simulink model "sedemo_rateestimator_withidlecomp"  (Simulink 7.5)
settings: Solver=VariableStepDiscrete  StartTime=0.0  StopTime=1200  MaxStep=inf  RelTol=1e-3
libraries: simeventssink1 x6, simeventstranslate1 x3, simeventsrouting1 x2, simeventstiming1 x2, simeventsgenerators1 x2, simeventsgates1 x1, simeventsqueue1 x1, simeventsinfo x1, simulink x1
settings Model: Creator=The MathWorks Inc.
settings DataIOCC: SaveOutput=off  SaveTime=off
settings OptimizationCC: InitFltsAndDblsToZero=on  EfficientMapNaN2IntZero=off
settings DebuggingCC: AlgebraicLoopMsg=error  SolverPrmCheckMsg=none  StrictBusMsg=Warning
settings SimEventsCC: propDiagAttribOutput=1  propDiagFcnCallOutput=1  propDiagStatOutput=0

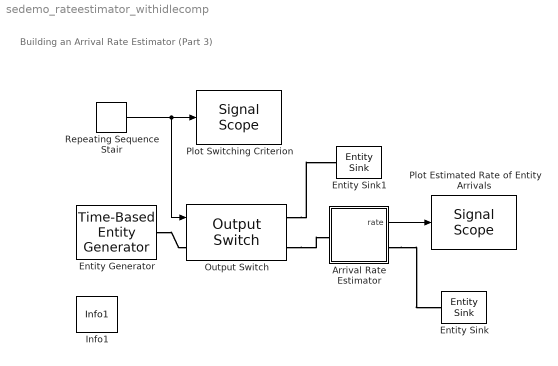
== system sedemo_rateestimator_withidlecomp ==
  note: Building an Arrival Rate Estimator (Part 3)
  Arrival Rate Estimator : Subsystem  mask(Rate Estimator){p=0.1, t_def=30}
      mask prompts: p "Smoothing factor p (0<p<1):"; t_def "Default sampling interval:"
      mask help:
      | Estimate number of arriving entities per second, where p is a smoothing factor that determines how much weight is given to the old estimate. If p is near 0, the estimate is more sensitive. If p is near 1, the estimate is smoother.
      |
      | The default sampling interval indicates the period of rate estimation computations during idle intervals when no entities arrive.
  Entity Generator : simeventsgenerators1/Entity Generators/Time-Based Entity Generator  Priority=1  DialogController=des_ddg_create  DialogControllerArgs=DataTag13  SystemSampleTime=-1  GenerateEntitiesUpon=Intergeneration time from dialog  Distribution=Constant  Minimum=0  Maximum=1  Mean=1  InitialSeed=12345  Period=4  PriorityEntityGeneration=300  GenerateEntityAtSimulationStart=off  ResponseWhenBlocked=Pause generation  ResponseWhenUnblocked=Immediate restart  EntityType=Standard  StatNumberDeparted=Off  StatPendingEntity=Off  StatAverageIntergenerationTime=Off
      settings: AttributesFormatString=Period = %<Period>
  Entity Sink : simeventssink1/Entity Sink  Priority=1  SystemSampleTime=-1  AvailableForArrivals=on  StatNumberArrived=Off
  Entity Sink1 : simeventssink1/Entity Sink  Priority=1  SystemSampleTime=-1  AvailableForArrivals=on  StatNumberArrived=Off
  Info1 : simeventsinfo/Info1  SystemSampleTime=-1  file_name=sedemo_rateestimator_m
  Output Switch : simeventsrouting1/Output Switch  Priority=1  SystemSampleTime=-1  NumberOutputPorts=2  SwitchingCriterion=From signal port p  InitialSeed=34567  AttributeName=Attribute1  InitialConditionsOpt=on  InitialConditions=1  EntityBufferOpt=off  SpecifyEventPriority=off  PriorityOutputSwitchSelectPort=4100  TimeoutPortOpt=off  StatNumberDeparted=Off  StatNumberTimedOut=Off  StatPendingEntity=Off  StatLastDeparturePort=Off  EvaluatedNumPorts=2
  Plot Estimated Rate of Entity Arrivals : simeventssink1/Signal Scope  Priority=1  SystemSampleTime=-1  PlotType=Continuous  InputType=Signal  NumInputs=1  AttributeNameY=Count  XInputOptionSignal=Event time  XInputOptionEntity=Event time  AttributeNameX=Count  EnableEntityOutport=on  XMin=-3  XMax=1203  XLimitExceededOption=Stretch axis limits  YLimitExceededOption=Stretch axis limits  AxisGrid=on  AxisLegend=off  LineDisables=""  LineColors="0  0  1"  LineStyles=-  LineMarkers=.  OpenScopeAtSimStart=on  Title=Arrival Rate Estimated Upon Arrivals and During Idle Intervals  YLabel=""  XLabel=Time  FigurePosition=[517 203 438 210]  AxisZoom=off  DataStoreOption=Limited  DataPointsLimit=10000  StatNumberArrived=Off  ShowCountPlotted=off  ShowToolbar=on
      settings: YMin=-0.005  YMax=.3
  Plot Switching Criterion : simeventssink1/Signal Scope  Priority=1  SystemSampleTime=-1  PlotType=Stair  InputType=Signal  NumInputs=1  AttributeNameY=Count  XInputOptionSignal=Event time  XInputOptionEntity=Event time  AttributeNameX=Count  EnableEntityOutport=on  XMin=-3  XMax=1203  XLimitExceededOption=Stretch axis limits  YLimitExceededOption=Keep axis limits unchanged  AxisGrid=off  AxisLegend=off  LineDisables=""  LineColors="1  0  0"  LineStyles=-  LineMarkers=.  OpenScopeAtSimStart=off  Title=Switching Criterion (p=2 is through rate estimator)  YLabel=""  XLabel=Time  FigurePosition=[517 488 438 210]  AxisZoom=off  DataStoreOption=Limited  DataPointsLimit=10000  StatNumberArrived=Off  ShowCountPlotted=off  ShowToolbar=on
      settings: YMin=0.9  YMax=2.1
  Repeating Sequence Stair : simulink/Sources/Repeating Sequence Stair  SystemSampleTime=-1  OutValues=[2 1 2 1]  tsamp=200  OutMin=[]  OutMax=[]  OutDataTypeStr=float('double')  OutputDataTypeScalingMode=Specify via dialog  OutDataType=float('double')  ConRadixGroup=Best Precision: Vector-wise  OutScaling=2^-12
  wires:
  Arrival Rate Estimator/1(rate) -> Plot Estimated Rate of Entity Arrivals/1
  Repeating Sequence Stair/1 -> Output Switch/1, Plot Switching Criterion/1
  connections:
  Entity Generator/RConn1 -- Output Switch/LConn1
  Output Switch/RConn1 -- Entity Sink1/LConn1
  Output Switch/RConn2 -- Arrival Rate Estimator/LConn1
  Arrival Rate Estimator/RConn1 -- Entity Sink/LConn1

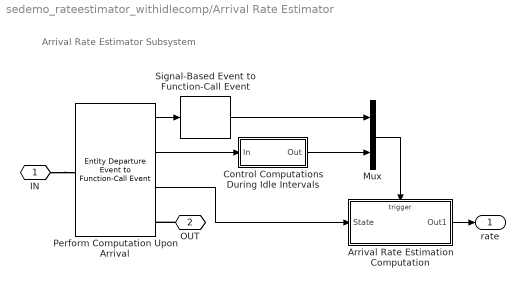
== system sedemo_rateestimator_withidlecomp/Arrival Rate Estimator ==
  note: Arrival Rate Estimator Subsystem
  Arrival Rate Estimation Computation : Subsystem  TreatAsAtomicUnit=on
      settings: PropExecContextOutsideSubsystem=on
  Control Computations During Idle Intervals : Subsystem
  Mux : Mux  Inputs=2
  Perform Computation Upon Arrival : simeventstranslate1/Entity Departure Event to Function-Call Event  Priority=1  SystemSampleTime=-1  TimingFunctionCallF1=After entity departure  EnableE1Port=off  EnableF2Port=on  TimingFunctionCallF2=After entity departure  EnableE2Port=off  StatNumberDeparted=Off  StatNumberF1Calls=On  StatNumberF2Calls=Off  IsInsideAFB=off
  Signal-Based Event to Function-Call Event : simeventstranslate1/Signal-Based Event to Function-Call Event  Priority=1  SystemSampleTime=-1  GenerateFunctionCallUpon=Function call from port fcn  SignalEdgeOption=Rising  EnableE1Port=off  EnableF2Port=off  EnableE2Port=off  SpecifyEventPriority=on  PriorityFunctionCall=2000  FunctionCallDelayFrom=Dialog  DelayFunctionCall=0  StatNumberF1Calls=Off  StatNumberF2Calls=Off  MaskBlockType=none
  IN : PMIOPort  Port=1  Side=Left
  OUT : PMIOPort  Port=2  Side=Right
  rate : Outport  OutDataType=sfix(16)  OutScaling=2^0
  wires:
  Arrival Rate Estimation Computation/1(Out1) -> rate/1
  Mux/1 -> Arrival Rate Estimation Computation/Trigger
  Perform Computation Upon Arrival/2 -> Control Computations During Idle Intervals/1(In)
  Control Computations During Idle Intervals/1(Out) -> Mux/2
  Perform Computation Upon Arrival/1 -> Signal-Based Event to Function-Call Event/1
  Perform Computation Upon Arrival/3 -> Arrival Rate Estimation Computation/1(State)
  Signal-Based Event to Function-Call Event/1 -> Mux/1
  connections:
  IN/RConn1 -- Perform Computation Upon Arrival/LConn1
  OUT/RConn1 -- Perform Computation Upon Arrival/RConn1

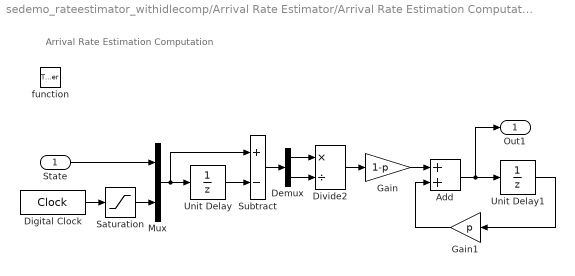
== system sedemo_rateestimator_withidlecomp/Arrival Rate Estimator/Arrival Rate Estimation Computation ==
  note: Arrival Rate Estimation Computation
  State : Inport  OutDataType=sfix(16)  OutScaling=2^0
  function : TriggerPort  TriggerType=function-call
  Add : Sum  OutDataType=sfix(16)  OutScaling=2^-10
  Demux : Demux  Outputs=2
  Digital Clock : DigitalClock  SampleTime=-1
  Divide2 : Product  Inputs=*/  OutDataType=sfix(16)  OutScaling=2^-10
  Gain : Gain  Gain=1-p  ParameterDataType=sfix(16)  ParameterScaling=2^0  OutDataType=sfix(16)  OutScaling=2^0
  Gain1 : Gain  Gain=p  ParameterDataType=sfix(16)  ParameterScaling=2^0  OutDataType=sfix(16)  OutScaling=2^0
  Mux : Mux  Inputs=2
  Saturation : Saturate  UpperLimit=inf  LowerLimit=1e-5  ZeroCross=off  OutDataType=sfix(16)  OutScaling=2^0
  Subtract : Sum  Inputs=+-  OutDataType=sfix(16)  OutScaling=2^-10
  Unit Delay : UnitDelay  SampleTime=-1
  Unit Delay1 : UnitDelay  SampleTime=-1
  Out1 : Outport  OutDataType=sfix(16)  OutScaling=2^0
  wires:
  Saturation/1 -> Mux/2
  Mux/1 -> Subtract/1, Unit Delay/1
  Digital Clock/1 -> Saturation/1
  Demux/2 -> Divide2/2
  Demux/1 -> Divide2/1
  Gain/1 -> Add/1
  State/1 -> Mux/1
  Unit Delay/1 -> Subtract/2
  Unit Delay1/1 -> Gain1/1
  Gain1/1 -> Add/2
  Add/1 -> Unit Delay1/1, Out1/1
  Divide2/1 -> Gain/1
  Subtract/1 -> Demux/1

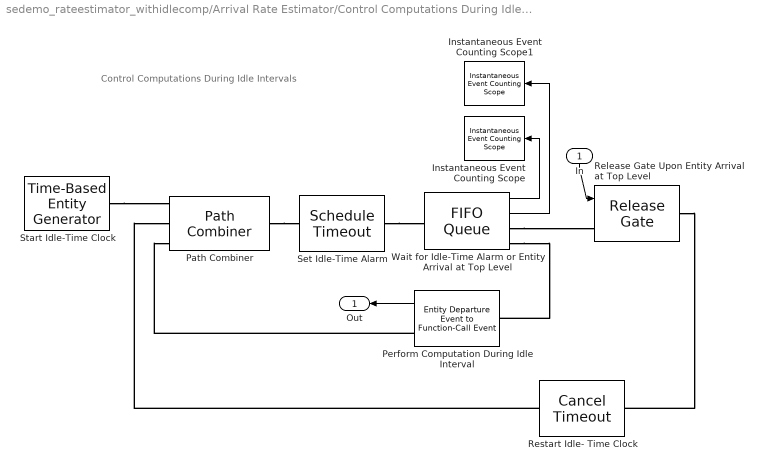
== system sedemo_rateestimator_withidlecomp/Arrival Rate Estimator/Control Computations During Idle Intervals ==
  note: Control Computations
      | During Idle Intervals
  In : Inport
  Instantaneous Event Counting Scope : simeventssink1/Instantaneous Event Counting Scope  Priority=1  SystemSampleTime=-1  PlotType=Instantaneous event counting  InputType=Signal  NumInputs=1  AttributeNameY=Count  XInputOptionSignal=Event time  XInputOptionEntity=Event time  AttributeNameX=Count  EnableEntityOutport=on  XMin=0  XMax=605  XLimitExceededOption=Stretch axis limits  YLimitExceededOption=Stretch axis limits  AxisGrid=on  AxisLegend=off  LineDisables=""  LineColors=b  LineStyles=-  LineMarkers=.  OpenScopeAtSimStart=off  Title=Computations Based on Entity Arrivals  YLabel=Number of Events  XLabel=Time  FigurePosition=[84 574 438 136]  AxisZoom=off  DataStoreOption=Limited  DataPointsLimit=10000  StatNumberArrived=Off  ShowCountPlotted=off  PlotPointsUpon=Change in signal from port vc  ChangeType=Rising  ShowToolbar=on
      settings: YMin=0  YMax=2
  Instantaneous Event Counting Scope1 : simeventssink1/Instantaneous Event Counting Scope  Priority=1  SystemSampleTime=-1  PlotType=Instantaneous event counting  InputType=Signal  NumInputs=1  AttributeNameY=Count  XInputOptionSignal=Event time  XInputOptionEntity=Event time  AttributeNameX=Count  EnableEntityOutport=on  XMin=0  XMax=605  XLimitExceededOption=Stretch axis limits  YLimitExceededOption=Stretch axis limits  AxisGrid=on  AxisLegend=off  LineDisables=""  LineColors=b  LineStyles=-  LineMarkers=.  OpenScopeAtSimStart=off  Title=Computations During Idle Intervals  YLabel=Number of Events  XLabel=Time  FigurePosition=[530 572 438 136]  AxisZoom=off  DataStoreOption=Limited  DataPointsLimit=10000  StatNumberArrived=Off  ShowCountPlotted=off  PlotPointsUpon=Change in signal from port vc  ChangeType=Rising  ShowToolbar=on
      settings: YMin=0  YMax=2
  Path Combiner : simeventsrouting1/Path Combiner  Priority=1  SystemSampleTime=-1  NumberInputPorts=3  InputPortPrecedence=IN1 port  InitialSeed=45675  SpecifyEventPriority=off  PriorityPathCombinerPortPrecedenceSelection=4100  StatNumberDeparted=Off  StatLastArrivalPort=Off  EvaluatedNumPorts=3
  Perform Computation During Idle Interval : simeventstranslate1/Entity Departure Event to Function-Call Event  Priority=1  SystemSampleTime=-1  TimingFunctionCallF1=After entity departure  EnableE1Port=off  EnableF2Port=off  TimingFunctionCallF2=After entity departure  EnableE2Port=off  StatNumberDeparted=Off  StatNumberF1Calls=Off  StatNumberF2Calls=Off  IsInsideAFB=off
  Release Gate Upon Entity Arrival at Top Level : simeventsgates1/Release Gate  Priority=1  SystemSampleTime=-1  OpenGateUpon=Function call from port fcn  SignalEdgeOption=Rising  SpecifyEventPriority=off  PriorityGateRelease=2200  StatNumberDeparted=Off
  Restart Idle- Time Clock : simeventstiming1/Cancel Timeout  Priority=0  SystemSampleTime=-1  TimeoutTag=TO1  TimeoutModeOption=Continue  TimeoutCancelledOption=Error  StatNumberDeparted=Off  StatTimeoutNumberDeparted=Off  StatResidualTimeout=Off  StatAverageResidualTimeout=Off
  Set Idle-Time Alarm : simeventstiming1/Schedule Timeout  Priority=0  SystemSampleTime=-1  TimeoutTag=TO1  TimeoutIntervalFrom=Dialog  TimeoutInterval=t_def  AttributeName=TimeoutAttribute  PriorityTimeout=1700  TimeoutScheduledOption=Error  TimeoutNoDestination=Error  StatNumberDeparted=Off
  Start Idle-Time Clock : simeventsgenerators1/Entity Generators/Time-Based Entity Generator  Priority=1  DialogController=des_ddg_create  DialogControllerArgs=DataTag8  SystemSampleTime=-1  GenerateEntitiesUpon=Intergeneration time from dialog  Distribution=Constant  Minimum=0  Maximum=1  Mean=1  InitialSeed=12345  Period=inf  PriorityEntityGeneration=300  GenerateEntityAtSimulationStart=on  ResponseWhenBlocked=Pause generation  ResponseWhenUnblocked=Immediate restart  EntityType=Blank  StatNumberDeparted=Off  StatPendingEntity=Off  StatAverageIntergenerationTime=Off
  Wait for Idle-Time Alarm or Entity Arrival at Top Level : simeventsqueue1/FIFO Queue  Priority=1  SystemSampleTime=-1  Capacity=2  EnableTOPort=on  StatNumberDeparted=On  StatNumberInBlock=Off  StatPendingEntity=Off  StatAverageWait=Off  StatAverageQueueLength=Off  StatNumberTimedout=On
  Out : Outport
  wires:
  Wait for Idle-Time Alarm or Entity Arrival at Top Level/2 -> Instantaneous Event Counting Scope1/1
  Wait for Idle-Time Alarm or Entity Arrival at Top Level/1 -> Instantaneous Event Counting Scope/1
  In/1 -> Release Gate Upon Entity Arrival at Top Level/1
  Perform Computation During Idle Interval/1 -> Out/1
  connections:
  Start Idle-Time Clock/RConn1 -- Path Combiner/LConn1
  Path Combiner/RConn1 -- Set Idle-Time Alarm/LConn1
  Wait for Idle-Time Alarm or Entity Arrival at Top Level/RConn2 -- Perform Computation During Idle Interval/LConn1
  Perform Computation During Idle Interval/RConn1 -- Path Combiner/LConn3
  Wait for Idle-Time Alarm or Entity Arrival at Top Level/RConn1 -- Release Gate Upon Entity Arrival at Top Level/LConn1
  Release Gate Upon Entity Arrival at Top Level/RConn1 -- Restart Idle- Time Clock/LConn1
  Restart Idle- Time Clock/RConn1 -- Path Combiner/LConn2
  Set Idle-Time Alarm/RConn1 -- Wait for Idle-Time Alarm or Entity Arrival at Top Level/LConn1
